simulink model "monocykl3"  (R2023b)
settings: Solver=FixedStepAuto  StartTime=0.0  StopTime=120  FixedStep=0.01  RelTol=1e-3
undefined symbols (not defined in the file or in its folder): tau
libraries: slpidlib x1
settings Model: Creator=student  LastModifiedBy=Admin
settings OptimizationCC: BlockReduction=off  DefaultParameterBehavior=Inlined  BufferReuse=off

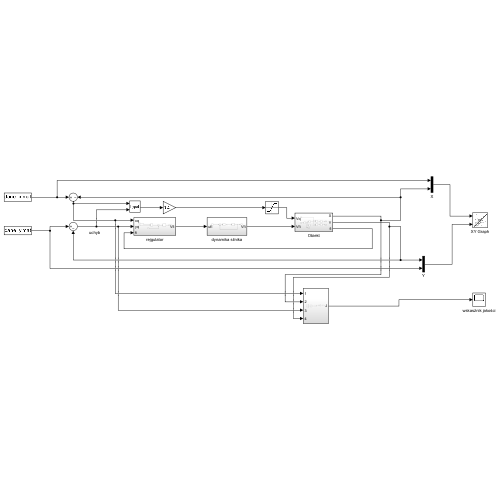
[thumbnail: Simulink's stored preview of the top-level diagram]
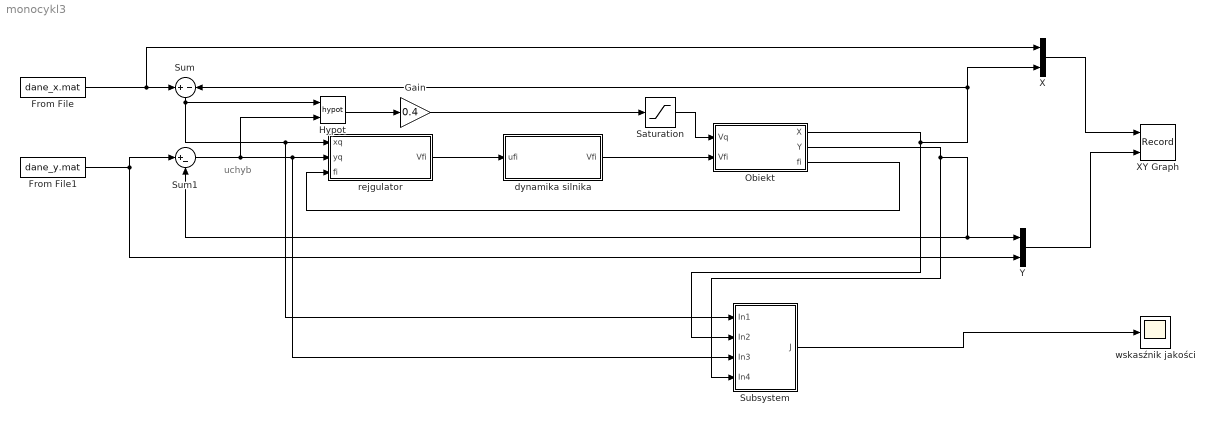
== system monocykl3 ==
  note: uchyb
  From File : FromFile  FileName=dane_x.mat  SampleTime=0  ExtrapolationAfterLastDataPoint=Hold last value
  From File1 : FromFile  FileName=dane_y.mat  SampleTime=0  ExtrapolationAfterLastDataPoint=Hold last value
  Gain : Gain  Gain=0.4
  Hypot : Math  Operator=hypot
  Obiekt : Subsystem
  Saturation : Saturate  UpperLimit=10  LowerLimit=-10
  Subsystem : Subsystem
  Sum : Sum  Inputs=+|-
  Sum1 : Sum  Inputs=|+-
  X : Mux  Inputs=2
  XY Graph : Record  FileSettingsInternal="{\"entries\":[{\"content\":{\"excelSettings\":{\"content\":{},\"type\":\"Streamout.ExcelSettings\"}},\"type\":\"Streamout.FileSettingStorage\",\"uuid\":\"\"}],\"packageUris\":[\"http:\\/\\/schema.mathworks.com\\/mf0\\/streamout_blocks\\/R2020a\"],\"version\":\"1.0\"}"  Layout=[1 1]  SignalsInternal="{\"entries\":[{\"content\":{\"signals\":[{\"content\":{\"blockPath\":[],\"dimensions\":[2],\"domain\":\"\",\"hasChildren\":true,\"lineColor\":\"#64d413\",\"port\":1,\"signalID\":887,\"signalName\":\"X\"},\"type\":\"RecordBlkView.Signal\",\"uuid\":\"\"},{\"content\":{\"blockPath\":[],\"channel\":[1],\"dimensions\":[2],\"domain\":\"\",\"lineColor\":\"#139fff\",\"parentID\":887,\"plots\":[1],\"port\":1,\"signalID\":888,\"signalName\":\"X\"},\"type\":\"RecordBlkView.Signal\",\"uuid\":\"\"},{\"content\":{\"blockPath\":[],\"channel\":[2],\"dimensions\":[2],\"domain\":\"\",\"lineColor\":\"#64d413\",\"parentID\":887,\"plots\":[1],\"port\":1,\"signalID\":889,\"signalName\":\"X\"},\"type\":\"RecordBlkView.Signal\",\"uuid\":\"\"},{\"content\":{\"blockPath\":[],\"dimensions\":[2],\"domain\":\"\",\"hasChildren\":true,\"lineColor\":\"#fe330a\",\"port\":2,\"signalID\":894,\"signalName\":\"Y\"},\"type\":\"RecordBlkView.Signal\",\"uuid\":\"\"},{\"content\":{\"blockPath\":[],\"channel\":[1],\"dimensions\":[2],\"domain\":\"\",\"lineColor\":\"#b746ff\",\"parentID\":894,\"plots\":[1],\"port\":2,\"signalID\":895,\"signalName\":\"Y\"},\"type\":\"RecordBlkView.Signal\",\"uuid\":\"\"},{\"content\":{\"blockPath\":[],\"channel\":[2],\"dimensions\":[2],\"domain\":\"\",\"lineColor\":\"#ff13a6\",\"parentID\":894,\"plots\":[1],\"port\":2,\"signalID\":896,\"signalName\":\"Y\"},\"type\":\"RecordBlkView.Signal\",\"uuid\":\"\"}]},\"type\":\"RecordBlkView.InputSignals\",\"uuid\":\"\"}],\"packageUris\":[\"http:\\/\\/schema.mathworks.com\\/mf0\\/streamout_blocks\\/R2020a\"],\"version\":\"1.0\"}"  VisualizationBindings="{\"xyplotplugin\":{\"info\":[{\"series\":[{\"bindingParametersList\":[{\"parameter\":\"X-Axis\",\"signalID\":889,\"signalName\":\"X(2)\"},{\"parameter\":\"Y-Axis\",\"signalID\":895,\"signalName\":\"Y(1)\"}],\"seriesID\":50907},{\"bindingParametersList\":[{\"parameter\":\"X-Axis\",\"signalID\":888,\"signalName\":\"X(1)\"},{\"parameter\":\"Y-Axis\",\"signalID\":896,\"signalName\":\"Y(2)\"}],\"seriesID\":3662}],\"subplotID\":1}]}}"  CompatibilityTag=XY
  Y : Mux  Inputs=2
  dynamika silnika : Subsystem
  rejgulator : Subsystem
  wskasźnik jakości : Scope
  wires:
  Obiekt/2(Y) -> Subsystem/4(In4), Y/1, Sum1/2
  Obiekt/1(X) -> Subsystem/2(In2), X/2, Sum/2
  From File/1 -> X/1, Sum/1
  From File1/1 -> Y/2, Sum1/1
  Sum1/1 -> Subsystem/3(In3), rejgulator/2(yq), Hypot/2
  Sum/1 -> Subsystem/1(In1), rejgulator/1(xq), Hypot/1
  Y/1 -> XY Graph/2
  X/1 -> XY Graph/1
  Obiekt/3(fi) -> rejgulator/3(fi)
  Subsystem/1(J) -> wskasźnik jakości/1
  rejgulator/1(Vfi) -> dynamika silnika/1(ufi)
  Hypot/1 -> Gain/1
  Gain/1 -> Saturation/1
  Saturation/1 -> Obiekt/1(Vq)
  dynamika silnika/1(Vfi) -> Obiekt/2(Vfi)

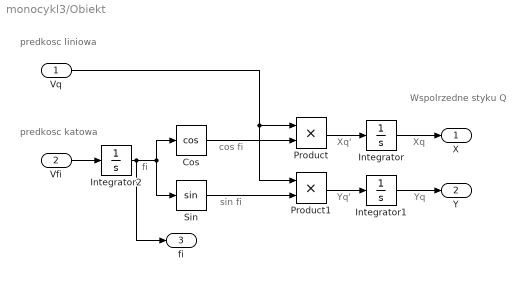
== system monocykl3/Obiekt ==
  note: Yq'
  note: Xq'
  note: sin fi
  note: cos fi
  note: fi
  note: Yq
  note: Xq
  note: Wspolrzedne styku Q
  note: predkosc katowa
  note: predkosc liniowa
  Vq : Inport
  Vfi : Inport  Port=2
  Cos : Trigonometry  Operator=cos
  Integrator : Integrator
  Integrator1 : Integrator
  Integrator2 : Integrator
  Product : Product
  Product1 : Product
  Sin : Trigonometry
  X : Outport
  Y : Outport  Port=2
  fi : Outport  Port=3
  wires:
  Integrator/1 -> X/1
  Integrator1/1 -> Y/1
  Vfi/1 -> Integrator2/1
  Integrator2/1 -> fi/1, Sin/1, Cos/1
  Vq/1 -> Product/1, Product1/1
  Product1/1 -> Integrator1/1
  Product/1 -> Integrator/1
  Sin/1 -> Product1/2
  Cos/1 -> Product/2

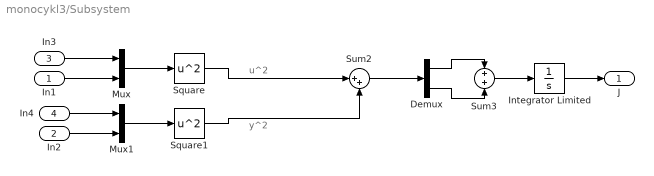
== system monocykl3/Subsystem ==
  note: y^2
  note: u^2
  In1 : Inport
  In2 : Inport  Port=2
  In3 : Inport  Port=3
  In4 : Inport  Port=4
  Demux : Demux  Outputs=2
  Integrator Limited : Integrator  LimitOutput=on  LowerSaturationLimit=0
  Mux : Mux  Inputs=2
  Mux1 : Mux  Inputs=2
  Square : Math  Operator=square
  Square1 : Math  Operator=square
  Sum2 : Sum  Inputs=|++
  Sum3 : Sum  Inputs=+|+
  J : Outport
  wires:
  Square1/1 -> Sum2/2
  Demux/1 -> Sum3/1
  Mux/1 -> Square/1
  Sum3/1 -> Integrator Limited/1
  In3/1 -> Mux/1
  Square/1 -> Sum2/1
  In2/1 -> Mux1/2
  Mux1/1 -> Square1/1
  Sum2/1 -> Demux/1
  Demux/2 -> Sum3/2
  In4/1 -> Mux1/1
  Integrator Limited/1 -> J/1
  In1/1 -> Mux/2

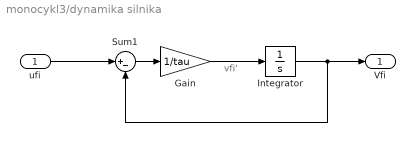
== system monocykl3/dynamika silnika ==
  note: vfi'
  ufi : Inport
  Gain : Gain  Gain=1/tau
  Integrator : Integrator
  Sum1 : Sum  Inputs=|+-
  Vfi : Outport
  wires:
  Sum1/1 -> Gain/1
  Gain/1 -> Integrator/1
  Integrator/1 -> Vfi/1, Sum1/2
  ufi/1 -> Sum1/1

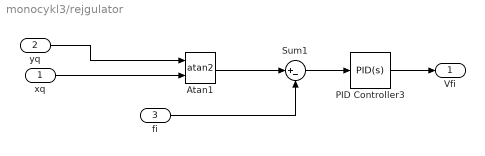
== system monocykl3/rejgulator ==
  xq : Inport
  yq : Inport  Port=2
  fi : Inport  Port=3
  Atan1 : Trigonometry  Operator=atan2
  PID Controller3 : slpidlib/PID Controller  Controller=PID  Form=Parallel  TimeDomain=Continuous-time  UseExternalTs=off  SampleTime=-1  IntegratorMethod=Forward Euler  FilterMethod=Forward Euler  ControllerParametersSource=internal  P=10  I=1  UseKiTs=off  D=0  N=100  UseFilter=on  TunerSelectOption=Transfer Function Based (PID Tuner App)  InitialConditionSource=internal  InitialConditionForIntegrator=0  InitialConditionForFilter=0  DifferentiatorICPrevScaledInput=0  ExternalReset=none  TrackingMode=off  Kt=1  LimitOutput=off  SatLimitsSource=internal  UpperSaturationLimit=inf  LowerSaturationLimit=-inf  LinearizeAsGain=on  AntiWindupMode=none  Kb=1  LimitIntegrator=off  UpperIntegratorSaturationLimit=inf  LowerIntegratorSaturationLimit=-inf  POutMin=[]  POutMax=[]  IOutMin=[]  IOutMax=[]  DOutMin=[]  DOutMax=[]  NOutMin=[]  NOutMax=[]  SumOutMin=[]  SumOutMax=[]  SaturationOutMin=[]  SaturationOutMax=[]  PParamMin=[]  PParamMax=[]  IParamMin=[]  IParamMax=[]  DParamMin=[]  DParamMax=[]  NParamMin=[]  NParamMax=[]  KbParamMin=[]  KbParamMax=[]  KtParamMin=[]  KtParamMax=[]  KbOutMin=[]  KbOutMax=[]  KtOutMin=[]  KtOutMax=[]  IntegratorOutMin=[]  IntegratorOutMax=[]  FilterOutMin=[]  FilterOutMax=[]  SumI1OutMin=[]  SumI1OutMax=[]  SumI2OutMin=[]  SumI2OutMax=[]  SumI3OutMin=[]  SumI3OutMax=[]  SumI4OutMin=[]  SumI4OutMax=[]  SumDOutMin=[]  SumDOutMax=[]  DifferentiatorOutMin=[]  DifferentiatorOutMax=[]  FilterDiffOutCoefMin=[]  FilterDiffOutCoefMax=[]  ReciprocalOutMin=[]  ReciprocalOutMax=[]  SumDenOutMin=[]  SumDenOutMax=[]  SumNumOutMin=[]  SumNumOutMax=[]  DivideOutMin=[]  DivideOutMax=[]  UdiffTsProdOutMin=[]  UdiffTsProdOutMax=[]  NTsProdOutMin=[]  NTsProdOutMax=[]  UintegralTsProdOutMin=[]  UintegralTsProdOutMax=[]  UngainTsProdOutMin=[]  UngainTsProdOutMax=[]  ClampingZeroOutDataTypeStr=Inherit: Inherit via back propagation  ClampingZeroOutMin=[]  ClampingZeroOutMax=[]  FilterDenConstantOutDataTypeStr=Inherit: Inherit via back propagation  FilterDenConstantOutMin=[]  FilterDenConstantOutMax=[]  PCopyOutDataTypeStr=Inherit: Inherit via back propagation  PCopyOutMin=[]  PCopyOutMax=[]  NCopyOutDataTypeStr=Inherit: Inherit via back propagation  NCopyOutMin=[]  NCopyOutMax=[]  IntegratorContinuousStateAttributes=''  IntegratorStateMustResolveToSignalObject=off  IntegratorRTWStateStorageClass=Auto  FilterContinuousStateAttributes=''  FilterStateMustResolveToSignalObject=off  FilterRTWStateStorageClass=Auto  ParallelPVariant=InternalParameters  IdealPVariant=Disabled  IVariant=InternalParameters  DVariant=InternalParameters  IntegratorVariant=Continuous  SatVariant=Disabled  AWVariant=Passthrough  PCopyVariant=Disabled  TRVariant=Disabled  FdbkBlocksVariant=Forward  IdealPFdbkVariant=Disabled  SatFdbkVariant=Disabled  DerivativeFilterVariant=ContFilter  NVariant=InternalParameters  NCopyVariant=Disabled  FilterICVariant=InternalICsFilter  IntegratorICVariant=InternalICs  ExternalResetVariant=Disabled  TRSumVariant=Passthrough  SumFdbkVariant=Disabled  SumVariant=Sum_PID  TsampFilterVariant=InternalTs  TsampNgainVariant=Passthrough  TsampIntegralVariant=Disabled_SignalSpec  ExternalSaturationOutDataTypeStr=Inherit: Same as second input
  Sum1 : Sum  Inputs=|+-
  Vfi : Outport
  wires:
  yq/1 -> Atan1/1
  xq/1 -> Atan1/2
  Atan1/1 -> Sum1/1
  fi/1 -> Sum1/2
  Sum1/1 -> PID Controller3/1
  PID Controller3/1 -> Vfi/1
